simulink model "gap_generation_platoon"  (R2019a)
settings: Solver=VariableStepAuto  StartTime=0.0  StopTime=50  RelTol=1e-3
libraries: simulink x68, powerlib_meascontrol x7, autolibshared x7
(part 1 of 3)
settings Model: Creator=fvall  LastModifiedBy=fvall

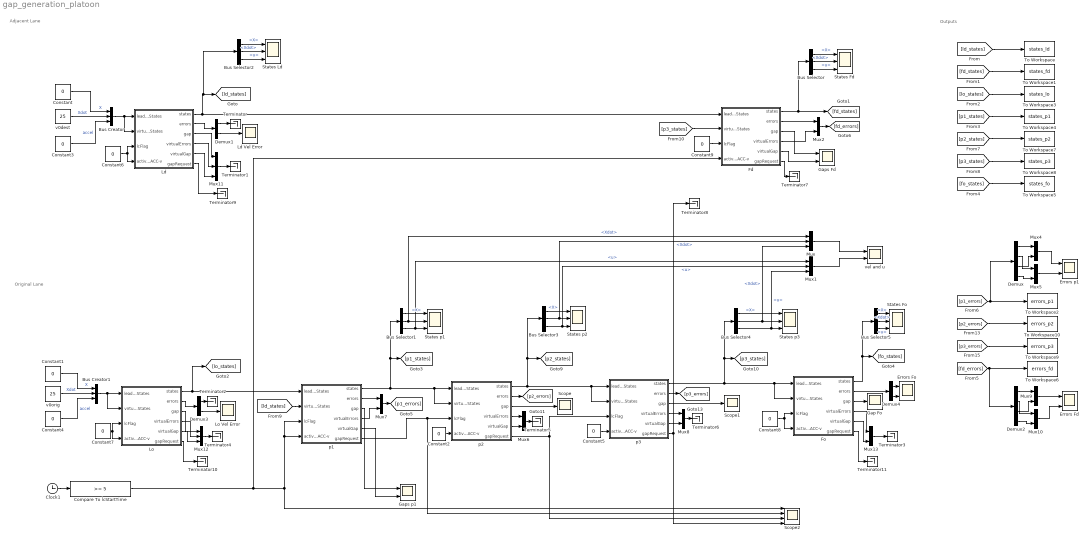
== system gap_generation_platoon ==
  note: Original Lane
  note: Adjacent Lane
  note: Outputs
  Bus Creator : BusCreator  Inputs=3
  Bus Creator1 : BusCreator  Inputs=3
  Bus Selector{,1..5} (6 alike) : BusSelector  OutputSignals=X,Xdot,u
  Clock1 : Clock
  Compare To lcStartTime : simulink/Logic and Bit Operations/Compare To Constant  relop=>=  const=5  OutDataTypeStr=boolean
  Constant{,1..9} (10 alike) : Constant  Value=0
  Demux : Demux
  Demux1 : Demux  Outputs=2
  Demux2 : Demux
  Demux3 : Demux  Outputs=2
  Demux4 : Demux  Outputs=2
  Errors Fd : Scope  NumInputPorts=2
  Errors Fo : Scope  NumInputPorts=2
  Errors p1 : Scope  NumInputPorts=2
  Fd : Subsystem  mask{m=2000, lf=2.5, lr=2.5, maxAcceleration=4, minAcceleration=-8, maxJerk=50, minJerk=-50, x0=62.7512, vx0=25, y0=3.6, h=0.63, hLc=2.215, d0=0.5004, d0Lc=0.5004, minHeadwayError=-100, maxHeadwayError=3, velFilterGain=10, Kd=1.5652, Kp=2.2775, Ki=0.75, velKi=0.5, velKp=1.5, vMin=18, hFilterGain=1, l1=-2}
      mask prompts: m "autoblks_shared:autoblkVehBody3DofLat:blkPrm_m"; lf "autoblks_shared:autoblkVehBody3DofLat:blkPrm_a"; lr "autoblks_shared:autoblkVehBody3DofLat:blkPrm_b"; maxAcceleration "Max Acceleration"; minAcceleration "Min Acceleration"; maxJerk "Max Jerk"; minJerk "Min Jerk"; x0 "autoblks_shared:autoblkVehBody3DofLat:blkPrm_X_o"; vx0 "autoblks_shared:autoblkVehBody3DofLat:blkPrm_xdot_o"; y0 "autoblks_shared:autoblkVehBody3DofLat:blkPrm_Y_o"; h "Time Headway"; hLc "Time Headway LC"; d0 "Standstill Gap"; d0Lc "Standstill Gap LC"; minHeadwayError "Min Headway Error"; maxHeadwayError "Max Headway Error"; velFilterGain "Velocity Filter Gain"; vMin "Min Gap Gen Speed"; hFilterGain "Headway filter Gain"; l1 "ACC-v Headway Error Threshold"
      mask TypeOptions m: Vehicle Body 3DOF Single Track/m
      mask TypeOptions lf: Vehicle Body 3DOF Single Track/a
      mask TypeOptions lr: Vehicle Body 3DOF Single Track/b
      mask TypeOptions x0: Vehicle Body 3DOF Single Track/X_o
      mask TypeOptions vx0: Vehicle Body 3DOF Single Track/xdot_o
      mask TypeOptions y0: Vehicle Body 3DOF Single Track/Y_o
      mask TypeOptions h: ACC/Headway error/h/Value
      mask TypeOptions hLc: ACC/Headway error/hLc/Value
      mask TypeOptions d0: ACC/Headway error/d0/Value
      mask TypeOptions d0Lc: ACC/Headway error/d0Lc/Value
      mask TypeOptions Kd: ACC/Kd/Gain
      mask TypeOptions Kp: ACC/Kp/Gain
      mask TypeOptions Ki: ACC/Ki/Gain
      mask TypeOptions velKi: ACC/velKi/Gain
      mask TypeOptions velKp: ACC/velKp/Gain
      mask TypeOptions vMin: ACC-v/vMin/Value
      mask TypeOptions hFilterGain: ACC/Headway error/hFilterGain/Gain
      mask TypeOptions l1:
      | ACC-v/Compare
      | To Constant/const
      mask DialogControl DescGroupVar Prompt: 3DOF Vehicle with ACC
      mask DialogControl DescTextVar Prompt: Vehicle with ACC. The vehicle model is Simulink's 3DOF single track vehicle body. The controller is a PID with constant headway including headway error saturation and filtered leader velocity.
      mask DialogControl ParameterGroupVar Prompt: Vehicle Parameters
      mask DialogControl m Prompt: Vehicle mass, m [kg]:
      mask DialogControl lf Prompt: Longitudinal distance from center of mass to front axle, a [m]:
      mask DialogControl lr Prompt: Longitudinal distance from center of mass to rear axle, b [m]:
      mask DialogControl x0 Prompt: Initial inertial frame longitudinal position, X_o [m]:
      mask DialogControl vx0 Prompt: Initial longitudinal velocity, xdot_o [m/s]:
      mask DialogControl y0 Prompt: Initial inertial frame lateral displacement, Y_o [m]:
      mask DialogControl Container3 Prompt: Controller Parameters
  Fo : Subsystem  mask{m=2000, lf=2.5, lr=2.5, maxAcceleration=4, minAcceleration=-8, maxJerk=50, minJerk=-50, x0=0, vx0=25, y0=0, h=0.63, hLc=2.215, d0=0.5004, d0Lc=0.5004, minHeadwayError=-100, maxHeadwayError=3, velFilterGain=10, Kd=1.5652, Kp=2.2775, Ki=0.75, velKi=0.5, velKp=1.5, vMin=18, hFilterGain=1, l1=-2}
      mask prompts: m "autoblks_shared:autoblkVehBody3DofLat:blkPrm_m"; lf "autoblks_shared:autoblkVehBody3DofLat:blkPrm_a"; lr "autoblks_shared:autoblkVehBody3DofLat:blkPrm_b"; maxAcceleration "Max Acceleration"; minAcceleration "Min Acceleration"; maxJerk "Max Jerk"; minJerk "Min Jerk"; x0 "autoblks_shared:autoblkVehBody3DofLat:blkPrm_X_o"; vx0 "autoblks_shared:autoblkVehBody3DofLat:blkPrm_xdot_o"; y0 "autoblks_shared:autoblkVehBody3DofLat:blkPrm_Y_o"; h "Time Headway"; hLc "Time Headway LC"; d0 "Standstill Gap"; d0Lc "Standstill Gap LC"; minHeadwayError "Min Headway Error"; maxHeadwayError "Max Headway Error"; velFilterGain "Velocity Filter Gain"; vMin "Min Gap Gen Speed"; hFilterGain "Headway filter Gain"; l1 "ACC-v Headway Error Threshold"
      mask TypeOptions m: Vehicle Body 3DOF Single Track/m
      mask TypeOptions lf: Vehicle Body 3DOF Single Track/a
      mask TypeOptions lr: Vehicle Body 3DOF Single Track/b
      mask TypeOptions x0: Vehicle Body 3DOF Single Track/X_o
      mask TypeOptions vx0: Vehicle Body 3DOF Single Track/xdot_o
      mask TypeOptions y0: Vehicle Body 3DOF Single Track/Y_o
      mask TypeOptions h: ACC/Headway error/h/Value
      mask TypeOptions hLc: ACC/Headway error/hLc/Value
      mask TypeOptions d0: ACC/Headway error/d0/Value
      mask TypeOptions d0Lc: ACC/Headway error/d0Lc/Value
      mask TypeOptions Kd: ACC/Kd/Gain
      mask TypeOptions Kp: ACC/Kp/Gain
      mask TypeOptions Ki: ACC/Ki/Gain
      mask TypeOptions velKi: ACC/velKi/Gain
      mask TypeOptions velKp: ACC/velKp/Gain
      mask TypeOptions vMin: ACC-v/vMin/Value
      mask TypeOptions hFilterGain: ACC/Headway error/hFilterGain/Gain
      mask TypeOptions l1:
      | ACC-v/Compare
      | To Constant/const
      mask DialogControl DescGroupVar Prompt: 3DOF Vehicle with ACC
      mask DialogControl DescTextVar Prompt: Vehicle with ACC. The vehicle model is Simulink's 3DOF single track vehicle body. The controller is a PID with constant headway including headway error saturation and filtered leader velocity.
      mask DialogControl ParameterGroupVar Prompt: Vehicle Parameters
      mask DialogControl m Prompt: Vehicle mass, m [kg]:
      mask DialogControl lf Prompt: Longitudinal distance from center of mass to front axle, a [m]:
      mask DialogControl lr Prompt: Longitudinal distance from center of mass to rear axle, b [m]:
      mask DialogControl x0 Prompt: Initial inertial frame longitudinal position, X_o [m]:
      mask DialogControl vx0 Prompt: Initial longitudinal velocity, xdot_o [m/s]:
      mask DialogControl y0 Prompt: Initial inertial frame lateral displacement, Y_o [m]:
      mask DialogControl Container3 Prompt: Controller Parameters
  Gap Fo : Scope
  Gaps Fd : Scope  NumInputPorts=2
  Gaps p1 : Scope  NumInputPorts=2
  Ld : Subsystem  mask{m=2000, lf=2.5, lr=2.5, maxAcceleration=4, minAcceleration=-8, maxJerk=50, minJerk=-50, x0=84.0016, vx0=25, y0=3.6, h=0.63, hLc=1.9025, d0=0.5004, d0Lc=0.5004, minHeadwayError=-100, maxHeadwayError=3, velFilterGain=10, Kd=1.5652, Kp=2.2775, Ki=0.75, velKi=0.5, velKp=1.5, vMin=18, hFilterGain=1, l1=-2}
      mask prompts: m "autoblks_shared:autoblkVehBody3DofLat:blkPrm_m"; lf "autoblks_shared:autoblkVehBody3DofLat:blkPrm_a"; lr "autoblks_shared:autoblkVehBody3DofLat:blkPrm_b"; maxAcceleration "Max Acceleration"; minAcceleration "Min Acceleration"; maxJerk "Max Jerk"; minJerk "Min Jerk"; x0 "autoblks_shared:autoblkVehBody3DofLat:blkPrm_X_o"; vx0 "autoblks_shared:autoblkVehBody3DofLat:blkPrm_xdot_o"; y0 "autoblks_shared:autoblkVehBody3DofLat:blkPrm_Y_o"; h "Time Headway"; hLc "Time Headway LC"; d0 "Standstill Gap"; d0Lc "Standstill Gap LC"; minHeadwayError "Min Headway Error"; maxHeadwayError "Max Headway Error"; velFilterGain "Velocity Filter Gain"; vMin "Min Gap Gen Speed"; hFilterGain "Headway filter Gain"; l1 "ACC-v Headway Error Threshold"
      mask TypeOptions m: Vehicle Body 3DOF Single Track/m
      mask TypeOptions lf: Vehicle Body 3DOF Single Track/a
      mask TypeOptions lr: Vehicle Body 3DOF Single Track/b
      mask TypeOptions x0: Vehicle Body 3DOF Single Track/X_o
      mask TypeOptions vx0: Vehicle Body 3DOF Single Track/xdot_o
      mask TypeOptions y0: Vehicle Body 3DOF Single Track/Y_o
      mask TypeOptions h: ACC/Headway error/h/Value
      mask TypeOptions hLc: ACC/Headway error/hLc/Value
      mask TypeOptions d0: ACC/Headway error/d0/Value
      mask TypeOptions d0Lc: ACC/Headway error/d0Lc/Value
      mask TypeOptions Kd: ACC/Kd/Gain
      mask TypeOptions Kp: ACC/Kp/Gain
      mask TypeOptions Ki: ACC/Ki/Gain
      mask TypeOptions velKi: ACC/velKi/Gain
      mask TypeOptions velKp: ACC/velKp/Gain
      mask TypeOptions vMin: ACC-v/vMin/Value
      mask TypeOptions hFilterGain: ACC/Headway error/hFilterGain/Gain
      mask TypeOptions l1:
      | ACC-v/Compare
      | To Constant/const
      mask DialogControl DescGroupVar Prompt: 3DOF Vehicle with ACC
      mask DialogControl DescTextVar Prompt: Vehicle with ACC. The vehicle model is Simulink's 3DOF single track vehicle body. The controller is a PID with constant headway including headway error saturation and filtered leader velocity.
      mask DialogControl ParameterGroupVar Prompt: Vehicle Parameters
      mask DialogControl m Prompt: Vehicle mass, m [kg]:
      mask DialogControl lf Prompt: Longitudinal distance from center of mass to front axle, a [m]:
      mask DialogControl lr Prompt: Longitudinal distance from center of mass to rear axle, b [m]:
      mask DialogControl x0 Prompt: Initial inertial frame longitudinal position, X_o [m]:
      mask DialogControl vx0 Prompt: Initial longitudinal velocity, xdot_o [m/s]:
      mask DialogControl y0 Prompt: Initial inertial frame lateral displacement, Y_o [m]:
      mask DialogControl Container3 Prompt: Controller Parameters
  Ld Vel Error : Scope
  Lo : Subsystem  mask{m=2000, lf=2.5, lr=2.5, maxAcceleration=4, minAcceleration=-8, maxJerk=50, minJerk=-50, x0=85.0016, vx0=25, y0=0, h=0.63, hLc=1.9025, d0=0.5004, d0Lc=0.5004, minHeadwayError=-100, maxHeadwayError=3, velFilterGain=10, Kd=1.5652, Kp=2.2775, Ki=0.75, velKi=0.5, velKp=1.5, vMin=18, hFilterGain=1, l1=-2}
      mask prompts: m "autoblks_shared:autoblkVehBody3DofLat:blkPrm_m"; lf "autoblks_shared:autoblkVehBody3DofLat:blkPrm_a"; lr "autoblks_shared:autoblkVehBody3DofLat:blkPrm_b"; maxAcceleration "Max Acceleration"; minAcceleration "Min Acceleration"; maxJerk "Max Jerk"; minJerk "Min Jerk"; x0 "autoblks_shared:autoblkVehBody3DofLat:blkPrm_X_o"; vx0 "autoblks_shared:autoblkVehBody3DofLat:blkPrm_xdot_o"; y0 "autoblks_shared:autoblkVehBody3DofLat:blkPrm_Y_o"; h "Time Headway"; hLc "Time Headway LC"; d0 "Standstill Gap"; d0Lc "Standstill Gap LC"; minHeadwayError "Min Headway Error"; maxHeadwayError "Max Headway Error"; velFilterGain "Velocity Filter Gain"; vMin "Min Gap Gen Speed"; hFilterGain "Headway filter Gain"; l1 "ACC-v Headway Error Threshold"
      mask TypeOptions m: Vehicle Body 3DOF Single Track/m
      mask TypeOptions lf: Vehicle Body 3DOF Single Track/a
      mask TypeOptions lr: Vehicle Body 3DOF Single Track/b
      mask TypeOptions x0: Vehicle Body 3DOF Single Track/X_o
      mask TypeOptions vx0: Vehicle Body 3DOF Single Track/xdot_o
      mask TypeOptions y0: Vehicle Body 3DOF Single Track/Y_o
      mask TypeOptions h: ACC/Headway error/h/Value
      mask TypeOptions hLc: ACC/Headway error/hLc/Value
      mask TypeOptions d0: ACC/Headway error/d0/Value
      mask TypeOptions d0Lc: ACC/Headway error/d0Lc/Value
      mask TypeOptions Kd: ACC/Kd/Gain
      mask TypeOptions Kp: ACC/Kp/Gain
      mask TypeOptions Ki: ACC/Ki/Gain
      mask TypeOptions velKi: ACC/velKi/Gain
      mask TypeOptions velKp: ACC/velKp/Gain
      mask TypeOptions vMin: ACC-v/vMin/Value
      mask TypeOptions hFilterGain: ACC/Headway error/hFilterGain/Gain
      mask TypeOptions l1:
      | ACC-v/Compare
      | To Constant/const
      mask DialogControl DescGroupVar Prompt: 3DOF Vehicle with ACC
      mask DialogControl DescTextVar Prompt: Vehicle with ACC. The vehicle model is Simulink's 3DOF single track vehicle body. The controller is a PID with constant headway including headway error saturation and filtered leader velocity.
      mask DialogControl ParameterGroupVar Prompt: Vehicle Parameters
      mask DialogControl m Prompt: Vehicle mass, m [kg]:
      mask DialogControl lf Prompt: Longitudinal distance from center of mass to front axle, a [m]:
      mask DialogControl lr Prompt: Longitudinal distance from center of mass to rear axle, b [m]:
      mask DialogControl x0 Prompt: Initial inertial frame longitudinal position, X_o [m]:
      mask DialogControl vx0 Prompt: Initial longitudinal velocity, xdot_o [m/s]:
      mask DialogControl y0 Prompt: Initial inertial frame lateral displacement, Y_o [m]:
      mask DialogControl Container3 Prompt: Controller Parameters
  Lo Vel Error : Scope
  Mux{,1,11..12} (4 alike) : Mux  Inputs=3
  Mux{2,4..10,13} (9 alike) : Mux  Inputs=2
  Scope : Scope
  Scope1 : Scope
  Scope2 : Scope  NumInputPorts=4
  States Fd : Scope  NumInputPorts=3
  States Fo : Scope  NumInputPorts=3
  States Ld : Scope  NumInputPorts=3
  States p1 : Scope  NumInputPorts=3
  States p2 : Scope  NumInputPorts=3
  States p3 : Scope  NumInputPorts=3
  Terminator{,1..11} (12 alike) : Terminator
  To Workspace : ToWorkspace  VariableName=states_ld  SampleTime=-1
  To Workspace1 : ToWorkspace  VariableName=states_fd  SampleTime=-1
  To Workspace10 : ToWorkspace  VariableName=errors_p2  SampleTime=-1
  To Workspace2 : ToWorkspace  VariableName=errors_p1  SampleTime=-1
  To Workspace3 : ToWorkspace  VariableName=states_lo  SampleTime=-1
  To Workspace4 : ToWorkspace  VariableName=states_p1  SampleTime=-1
  To Workspace5 : ToWorkspace  VariableName=states_fo  SampleTime=-1
  To Workspace6 : ToWorkspace  VariableName=errors_fd  SampleTime=-1
  To Workspace7 : ToWorkspace  VariableName=states_p2  SampleTime=-1
  To Workspace8 : ToWorkspace  VariableName=states_p3  SampleTime=-1
  To Workspace9 : ToWorkspace  VariableName=errors_p3  SampleTime=-1
  p1 : Subsystem  mask{m=2000, lf=2.5, lr=2.5, maxAcceleration=4, minAcceleration=-8, maxJerk=50, minJerk=-50, x0=63.7512, vx0=25, y0=0, h=0.63, hLc=2.215, d0=0.5004, d0Lc=0.5004, minHeadwayError=-100, maxHeadwayError=3, velFilterGain=10, Kd=1.5652, Kp=2.2775, Ki=0.75, velKi=0.5, velKp=1.5, vMin=18, hFilterGain=1, l1=-2}
      mask prompts: m "autoblks_shared:autoblkVehBody3DofLat:blkPrm_m"; lf "autoblks_shared:autoblkVehBody3DofLat:blkPrm_a"; lr "autoblks_shared:autoblkVehBody3DofLat:blkPrm_b"; maxAcceleration "Max Acceleration"; minAcceleration "Min Acceleration"; maxJerk "Max Jerk"; minJerk "Min Jerk"; x0 "autoblks_shared:autoblkVehBody3DofLat:blkPrm_X_o"; vx0 "autoblks_shared:autoblkVehBody3DofLat:blkPrm_xdot_o"; y0 "autoblks_shared:autoblkVehBody3DofLat:blkPrm_Y_o"; h "Time Headway"; hLc "Time Headway LC"; d0 "Standstill Gap"; d0Lc "Standstill Gap LC"; minHeadwayError "Min Headway Error"; maxHeadwayError "Max Headway Error"; velFilterGain "Velocity Filter Gain"; vMin "Min Gap Gen Speed"; hFilterGain "Headway filter Gain"; l1 "ACC-v Headway Error Threshold"
      mask TypeOptions m: Vehicle Body 3DOF Single Track/m
      mask TypeOptions lf: Vehicle Body 3DOF Single Track/a
      mask TypeOptions lr: Vehicle Body 3DOF Single Track/b
      mask TypeOptions x0: Vehicle Body 3DOF Single Track/X_o
      mask TypeOptions vx0: Vehicle Body 3DOF Single Track/xdot_o
      mask TypeOptions y0: Vehicle Body 3DOF Single Track/Y_o
      mask TypeOptions h: ACC/Headway error/h/Value
      mask TypeOptions hLc: ACC/Headway error/hLc/Value
      mask TypeOptions d0: ACC/Headway error/d0/Value
      mask TypeOptions d0Lc: ACC/Headway error/d0Lc/Value
      mask TypeOptions Kd: ACC/Kd/Gain
      mask TypeOptions Kp: ACC/Kp/Gain
      mask TypeOptions Ki: ACC/Ki/Gain
      mask TypeOptions velKi: ACC/velKi/Gain
      mask TypeOptions velKp: ACC/velKp/Gain
      mask TypeOptions vMin: ACC-v/vMin/Value
      mask TypeOptions hFilterGain: ACC/Headway error/hFilterGain/Gain
      mask TypeOptions l1:
      | ACC-v/Compare
      | To Constant/const
      mask DialogControl DescGroupVar Prompt: 3DOF Vehicle with ACC
      mask DialogControl DescTextVar Prompt: Vehicle with ACC. The vehicle model is Simulink's 3DOF single track vehicle body. The controller is a PID with constant headway including headway error saturation and filtered leader velocity.
      mask DialogControl ParameterGroupVar Prompt: Vehicle Parameters
      mask DialogControl m Prompt: Vehicle mass, m [kg]:
      mask DialogControl lf Prompt: Longitudinal distance from center of mass to front axle, a [m]:
      mask DialogControl lr Prompt: Longitudinal distance from center of mass to rear axle, b [m]:
      mask DialogControl x0 Prompt: Initial inertial frame longitudinal position, X_o [m]:
      mask DialogControl vx0 Prompt: Initial longitudinal velocity, xdot_o [m/s]:
      mask DialogControl y0 Prompt: Initial inertial frame lateral displacement, Y_o [m]:
      mask DialogControl Container3 Prompt: Controller Parameters
  p2 : Subsystem  mask{m=2000, lf=2.5, lr=2.5, maxAcceleration=4, minAcceleration=-8, maxJerk=50, minJerk=-50, x0=42.5008, vx0=25, y0=0, h=0.63, hLc=2.215, d0=0.5004, d0Lc=0.5004, minHeadwayError=-100, maxHeadwayError=3, velFilterGain=10, Kd=1.5652, Kp=2.2775, Ki=0.75, velKi=0.5, velKp=1.5, vMin=18, hFilterGain=1, l1=-2}
      mask prompts: m "autoblks_shared:autoblkVehBody3DofLat:blkPrm_m"; lf "autoblks_shared:autoblkVehBody3DofLat:blkPrm_a"; lr "autoblks_shared:autoblkVehBody3DofLat:blkPrm_b"; maxAcceleration "Max Acceleration"; minAcceleration "Min Acceleration"; maxJerk "Max Jerk"; minJerk "Min Jerk"; x0 "autoblks_shared:autoblkVehBody3DofLat:blkPrm_X_o"; vx0 "autoblks_shared:autoblkVehBody3DofLat:blkPrm_xdot_o"; y0 "autoblks_shared:autoblkVehBody3DofLat:blkPrm_Y_o"; h "Time Headway"; hLc "Time Headway LC"; d0 "Standstill Gap"; d0Lc "Standstill Gap LC"; minHeadwayError "Min Headway Error"; maxHeadwayError "Max Headway Error"; velFilterGain "Velocity Filter Gain"; vMin "Min Gap Gen Speed"; hFilterGain "Headway filter Gain"; l1 "ACC-v Headway Error Threshold"
      mask TypeOptions m: Vehicle Body 3DOF Single Track/m
      mask TypeOptions lf: Vehicle Body 3DOF Single Track/a
      mask TypeOptions lr: Vehicle Body 3DOF Single Track/b
      mask TypeOptions x0: Vehicle Body 3DOF Single Track/X_o
      mask TypeOptions vx0: Vehicle Body 3DOF Single Track/xdot_o
      mask TypeOptions y0: Vehicle Body 3DOF Single Track/Y_o
      mask TypeOptions h: ACC/Headway error/h/Value
      mask TypeOptions hLc: ACC/Headway error/hLc/Value
      mask TypeOptions d0: ACC/Headway error/d0/Value
      mask TypeOptions d0Lc: ACC/Headway error/d0Lc/Value
      mask TypeOptions Kd: ACC/Kd/Gain
      mask TypeOptions Kp: ACC/Kp/Gain
      mask TypeOptions Ki: ACC/Ki/Gain
      mask TypeOptions velKi: ACC/velKi/Gain
      mask TypeOptions velKp: ACC/velKp/Gain
      mask TypeOptions vMin: ACC-v/vMin/Value
      mask TypeOptions hFilterGain: ACC/Headway error/hFilterGain/Gain
      mask TypeOptions l1:
      | ACC-v/Compare
      | To Constant/const
      mask DialogControl DescGroupVar Prompt: 3DOF Vehicle with ACC
      mask DialogControl DescTextVar Prompt: Vehicle with ACC. The vehicle model is Simulink's 3DOF single track vehicle body. The controller is a PID with constant headway including headway error saturation and filtered leader velocity.
      mask DialogControl ParameterGroupVar Prompt: Vehicle Parameters
      mask DialogControl m Prompt: Vehicle mass, m [kg]:
      mask DialogControl lf Prompt: Longitudinal distance from center of mass to front axle, a [m]:
      mask DialogControl lr Prompt: Longitudinal distance from center of mass to rear axle, b [m]:
      mask DialogControl x0 Prompt: Initial inertial frame longitudinal position, X_o [m]:
      mask DialogControl vx0 Prompt: Initial longitudinal velocity, xdot_o [m/s]:
      mask DialogControl y0 Prompt: Initial inertial frame lateral displacement, Y_o [m]:
      mask DialogControl Container3 Prompt: Controller Parameters
  p3 : Subsystem  mask{m=2000, lf=2.5, lr=2.5, maxAcceleration=4, minAcceleration=-8, maxJerk=50, minJerk=-50, x0=21.2504, vx0=25, y0=0, h=0.63, hLc=2.215, d0=0.5004, d0Lc=0.5004, minHeadwayError=-100, maxHeadwayError=3, velFilterGain=10, Kd=1.5652, Kp=2.2775, Ki=0.75, velKi=0.5, velKp=1.5, vMin=18, hFilterGain=1, l1=-2}
      mask prompts: m "autoblks_shared:autoblkVehBody3DofLat:blkPrm_m"; lf "autoblks_shared:autoblkVehBody3DofLat:blkPrm_a"; lr "autoblks_shared:autoblkVehBody3DofLat:blkPrm_b"; maxAcceleration "Max Acceleration"; minAcceleration "Min Acceleration"; maxJerk "Max Jerk"; minJerk "Min Jerk"; x0 "autoblks_shared:autoblkVehBody3DofLat:blkPrm_X_o"; vx0 "autoblks_shared:autoblkVehBody3DofLat:blkPrm_xdot_o"; y0 "autoblks_shared:autoblkVehBody3DofLat:blkPrm_Y_o"; h "Time Headway"; hLc "Time Headway LC"; d0 "Standstill Gap"; d0Lc "Standstill Gap LC"; minHeadwayError "Min Headway Error"; maxHeadwayError "Max Headway Error"; velFilterGain "Velocity Filter Gain"; vMin "Min Gap Gen Speed"; hFilterGain "Headway filter Gain"; l1 "ACC-v Headway Error Threshold"
      mask TypeOptions m: Vehicle Body 3DOF Single Track/m
      mask TypeOptions lf: Vehicle Body 3DOF Single Track/a
      mask TypeOptions lr: Vehicle Body 3DOF Single Track/b
      mask TypeOptions x0: Vehicle Body 3DOF Single Track/X_o
      mask TypeOptions vx0: Vehicle Body 3DOF Single Track/xdot_o
      mask TypeOptions y0: Vehicle Body 3DOF Single Track/Y_o
      mask TypeOptions h: ACC/Headway error/h/Value
      mask TypeOptions hLc: ACC/Headway error/hLc/Value
      mask TypeOptions d0: ACC/Headway error/d0/Value
      mask TypeOptions d0Lc: ACC/Headway error/d0Lc/Value
      mask TypeOptions Kd: ACC/Kd/Gain
      mask TypeOptions Kp: ACC/Kp/Gain
      mask TypeOptions Ki: ACC/Ki/Gain
      mask TypeOptions velKi: ACC/velKi/Gain
      mask TypeOptions velKp: ACC/velKp/Gain
      mask TypeOptions vMin: ACC-v/vMin/Value
      mask TypeOptions hFilterGain: ACC/Headway error/hFilterGain/Gain
      mask TypeOptions l1:
      | ACC-v/Compare
      | To Constant/const
      mask DialogControl DescGroupVar Prompt: 3DOF Vehicle with ACC
      mask DialogControl DescTextVar Prompt: Vehicle with ACC. The vehicle model is Simulink's 3DOF single track vehicle body. The controller is a PID with constant headway including headway error saturation and filtered leader velocity.
      mask DialogControl ParameterGroupVar Prompt: Vehicle Parameters
      mask DialogControl m Prompt: Vehicle mass, m [kg]:
      mask DialogControl lf Prompt: Longitudinal distance from center of mass to front axle, a [m]:
      mask DialogControl lr Prompt: Longitudinal distance from center of mass to rear axle, b [m]:
      mask DialogControl x0 Prompt: Initial inertial frame longitudinal position, X_o [m]:
      mask DialogControl vx0 Prompt: Initial longitudinal velocity, xdot_o [m/s]:
      mask DialogControl y0 Prompt: Initial inertial frame lateral displacement, Y_o [m]:
      mask DialogControl Container3 Prompt: Controller Parameters
  v0dest : Constant  Value=25
  v0orig : Constant  Value=25
  vel and u : Scope  NumInputPorts=2
  wires:
  Clock1/1 -> Compare To lcStartTime/1
  Bus Selector3/3 -> Mux1/2, States p2/3  "<u>"
  Bus Selector3/2 -> Mux/2, States p2/2  "<Xdot>"
  Bus Selector3/1 -> States p2/1  "<X>"
  p2/1(states) -> p3/1(leaderStates), p3/2(virtualLeaderStates), [p2_states], Bus Selector3/1
  Bus Selector4/3 -> Mux1/3, States p3/3  "<u>"
  Bus Selector4/2 -> States p3/2, Mux/3  "<Xdot>"
  Bus Selector4/1 -> States p3/1  "<X>"
  p2/2(errors) -> [p2_errors]
  p3/2(errors) -> [p3_errors]
  [p2_errors] -> To Workspace10/1
  [p3_errors] -> To Workspace9/1
  Ld/2(errors) -> Demux1/1
  Bus Selector2/3 -> States Ld/3  "<u>"
  Fd/6(gapRequest) -> Terminator7/1
  Fd/4(virtualErrors) -> Mux2/2
  Fd/5(virtualGap) -> Gaps Fd/2
  Fd/1(states) -> Bus Selector/1, [fd_states]
  Ld/3(gap) -> Mux11/1
  Fd/3(gap) -> Gaps Fd/1
  Mux11/1 -> Terminator1/1
  Fd/2(errors) -> Mux2/1
  Demux1/2 -> Ld Vel Error/1
  Bus Selector2/2 -> States Ld/2  "<Xdot>"
  Bus Selector2/1 -> States Ld/1  "<X>"
  Ld/6(gapRequest) -> Terminator9/1
  Bus Selector/1 -> States Fd/1  "<X>"
  [p3_states] -> Fd/2(virtualLeaderStates)
  Constant9/1 -> Fd/3(lcFlag)
  Ld/5(virtualGap) -> Mux11/3
  Bus Selector/3 -> States Fd/3  "<u>"
  Constant6/1 -> Ld/3(lcFlag), Ld/4(activate ACC-v)
  Ld/4(virtualErrors) -> Mux11/2
  Bus Selector/2 -> States Fd/2  "<Xdot>"
  Ld/1(states) -> Fd/1(leaderStates), Bus Selector2/1, [ld_states]
  v0dest/1 -> Bus Creator/2  "Xdot"
  Constant3/1 -> Bus Creator/3  "accel"
  Mux2/1 -> [fd_errors]
  Constant/1 -> Bus Creator/1  "X"
  Demux1/1 -> Terminator/1
  Bus Creator/1 -> Ld/1(leaderStates), Ld/2(virtualLeaderStates)
  Lo/5(virtualGap) -> Mux12/3
  Lo/2(errors) -> Demux3/1
  Mux12/1 -> Terminator4/1
  Lo/3(gap) -> Mux12/1
  Lo/1(states) -> p1/1(leaderStates), [lo_states]
  Lo/6(gapRequest) -> Terminator10/1
  Demux3/1 -> Terminator2/1
  Bus Creator1/1 -> Lo/2(virtualLeaderStates), Lo/1(leaderStates)
  Lo/4(virtualErrors) -> Mux12/2
  Constant7/1 -> Lo/3(lcFlag), Lo/4(activate ACC-v)
  v0orig/1 -> Bus Creator1/2  "Xdot"
  Constant4/1 -> Bus Creator1/3  "accel"
  Constant1/1 -> Bus Creator1/1  "X"
  Demux3/2 -> Lo Vel Error/1
  Mux13/1 -> Terminator3/1
  Fo/2(errors) -> Demux4/1
  Fo/4(virtualErrors) -> Mux13/1
  Fo/6(gapRequest) -> Terminator11/1
  Fo/3(gap) -> Gap Fo/1
  Demux4/2 -> Errors Fo/2
  Constant8/1 -> Fo/3(lcFlag), Fo/4(activate ACC-v)
  Demux4/1 -> Errors Fo/1
  Fo/1(states) -> Bus Selector5/1, [fo_states]
  p3/1(states) -> Bus Selector4/1, [p3_states], Fo/1(leaderStates), Fo/2(virtualLeaderStates)
  Fo/5(virtualGap) -> Mux13/2
  p1/4(virtualErrors) -> Mux7/2
  p1/1(states) -> Bus Selector1/1, [p1_states], p2/2(virtualLeaderStates), p2/1(leaderStates)
  Bus Selector1/2 -> States p1/2, Mux/1  "<Xdot>"
  p1/5(virtualGap) -> Gaps p1/2
  Mux7/1 -> [p1_errors]
  Bus Selector1/1 -> States p1/1  "<X>"
  Compare To lcStartTime/1 -> Fd/4(activate ACC-v), Scope2/1, p1/3(lcFlag), p1/4(activate ACC-v)
  Bus Selector1/3 -> Mux1/1, States p1/3  "<u>"
  p1/2(errors) -> Mux7/1
  p1/3(gap) -> Gaps p1/1
  [ld_states] -> p1/2(virtualLeaderStates)
  p1/6(gapRequest) -> p2/3(lcFlag), Scope2/2
  p2/6(gapRequest) -> p3/3(lcFlag), Scope2/3
  p3/6(gapRequest) -> Terminator8/1, Scope2/4
  p2/4(virtualErrors) -> Mux6/1
  p2/5(virtualGap) -> Mux6/2
  Mux6/1 -> Terminator5/1
  p3/4(virtualErrors) -> Mux8/1
  Mux8/1 -> Terminator6/1
  p3/5(virtualGap) -> Mux8/2
  p2/3(gap) -> Scope/1
  p3/3(gap) -> Scope1/1
  [fd_states] -> To Workspace1/1
  [lo_states] -> To Workspace3/1
  Mux10/1 -> Errors Fd/2
  Mux4/1 -> Errors p1/1
  Demux/2 -> Mux5/1
  Mux9/1 -> Errors Fd/1
  Demux/3 -> Mux4/2
  Demux/1 -> Mux4/1
  Mux5/1 -> Errors p1/2
  Demux2/2 -> Mux10/1
  Demux2/3 -> Mux9/2
  [p1_errors] -> To Workspace2/1, Demux/1
  [fd_errors] -> Demux2/1, To Workspace6/1
  [p1_states] -> To Workspace4/1
  Demux2/4 -> Mux10/2
  [ld_states] -> To Workspace/1
  Demux/4 -> Mux5/2
  [fo_states] -> To Workspace5/1
  Demux2/1 -> Mux9/1
  [p2_states] -> To Workspace7/1
  [p3_states] -> To Workspace8/1
  Mux/1 -> vel and u/1
  Mux1/1 -> vel and u/2
  Constant2/1 -> p2/4(activate ACC-v)
  Constant5/1 -> p3/4(activate ACC-v)
  Bus Selector5/1 -> States Fo/1  "<X>"
  Bus Selector5/2 -> States Fo/2  "<Xdot>"
  Bus Selector5/3 -> States Fo/3  "<u>"

== system gap_generation_platoon/Fd ==
  leaderStates : Inport
  virtualLeaderStates : Inport  Port=2
  lcFlag : Inport  Port=3
  activate ACC-v : Inport  Port=4
  ACC : Subsystem
  ACC-v : Subsystem
  AND : Logic  Inputs=3  IconShape=distinctive  AllPortsSameDT=off  OutDataTypeStr=boolean
  Abs : Abs
  Abs1 : Abs  ZeroCross=off
  Bus Creator : BusCreator  Inputs=4
  Bus Selector : BusSelector  OutputSignals=InertFrm.RearAxl.Disp.X,InertFrm.RearAxl.Disp.Y,InertFrm.RearAxl.Vel.Xdot
  Compare To Constant : simulink/Logic and Bit Operations/Compare To Constant  relop=<=  const=0.5  OutDataTypeStr=boolean
  Compare To Constant1 : simulink/Logic and Bit Operations/Compare To Constant  relop=<=  const=0.5  OutDataTypeStr=boolean
  Constant : Constant  Value=0
  Constant1 : Constant  Value=maxAcceleration+1
  Gain : Gain  Gain=m/2
  Min : MinMax  Inputs=2
  Mux1 : Mux  Inputs=6
  On Delay : powerlib_meascontrol/Logic/On Delay  DelayType=On delay  delay=1  ic=0  Ts=0
      settings: SourceProductName=Simscape Electrical
  Scope : Scope  NumInputPorts=2
  Scope1 : Scope  NumInputPorts=3
  Signal Specification : SignalSpecification  Dimensions=1
  Switch : Switch  Criteria=u2 > Threshold
  Terminator : Terminator
  Transport Delay : TransportDelay
  Triggered Subsystem : Subsystem  TreatAsAtomicUnit=on
  Vehicle Body 3DOF Single Track : autolibshared/Vehicle Body 3DOF Single Track  trackMode=Single (bicycle)  inputMode=External longitudinal forces  frontSteerMode=on  rearSteerMode=off  windMode=off  muMode=off  extFMode=off  extMMode=off  extXo=off  extpsio=off  extxdoto=off  extro=off  extYo=off  extTamb=off  extydoto=off  aMode=2  NF=2  NR=2  m=m  a=lf  b=lr  h=0.35  X_o=x0  xdot_o=vx0  CalphaMode=off  sigmaMode=on  d=0  w=[1.4,1.4]  Cy_f=12e3  Cy_r=11e3  sigma_f=.1  sigma_r=.1  alpha_f_brk=[-.1 .1]  Cy_f_data=[-9e3 9e3]  alpha_r_brk=[-.1 .1]  Cy_r_data=[-9e3 9e3]  Y_o=y0  ydot_o=0  Izz=4000  psi_o=0  r_o=0  Af=2  Cd=.3  Cl=.1  Cpm=.1  beta_w=[0:0.01:0.3]  Cs=[0:0.03:0.9]  Cym=[0:0.01:0.3]  Pabs=101325  Tair=273  g=9.81  mu=1  xdot_tol=.01  Fznom=5000  Fxtire_sat=7e4  Fytire_sat=7e4  longOff=0  latOff=0  vertOff=0  wrapAng=off
      settings: SourceProductName=Powertrain Blockset  SourceProductBaseCode=PW
  states : Outport
  errors : Outport  Port=2
  gap : Outport  Port=3
  virtualErrors : Outport  Port=4
  virtualGap : Outport  Port=5
  gapRequest : Outport  Port=6
  wires:
  Bus Selector/3 -> Bus Creator/3  "<Xdot>"
  Bus Selector/1 -> Bus Creator/1  "<X>"
  Min/1 -> Scope1/3, Signal Specification/1  "u"
  ACC/1(u) -> Scope1/1, Min/1  "acc"
  Gain/1 -> Vehicle Body 3DOF Single Track/3, Vehicle Body 3DOF Single Track/2
  Constant/1 -> Vehicle Body 3DOF Single Track/1
  Vehicle Body 3DOF Single Track/1 -> Bus Selector/1
  Vehicle Body 3DOF Single Track/4 -> Mux1/3
  Vehicle Body 3DOF Single Track/3 -> Mux1/2
  Vehicle Body 3DOF Single Track/2 -> Mux1/1
  Vehicle Body 3DOF Single Track/5 -> Mux1/4
  Vehicle Body 3DOF Single Track/6 -> Mux1/5
  Vehicle Body 3DOF Single Track/7 -> Mux1/6
  Mux1/1 -> Terminator/1
  ACC/3(gap) -> gap/1
  Bus Creator/1 -> ACC/1(currentStates), ACC-v/1(currentStates), states/1
  leaderStates/1 -> ACC/2(leaderStates)
  virtualLeaderStates/1 -> ACC-v/2(leaderStates)
  ACC/2(errors) -> errors/1
  lcFlag/1 -> ACC-v/4(lcFlag), On Delay/1, ACC/3(lcFlag)
  Switch/1 -> Scope1/2, Min/2  "acc-v"
  ACC-v/1(u) -> Switch/1
  ACC-v/2(errors) -> virtualErrors/1
  ACC-v/3(gap) -> virtualGap/1
  Bus Selector/2 -> Bus Creator/2  "<Y>"
  Signal Specification/1 -> Transport Delay/1, Abs1/1, Bus Creator/4, Gain/1
  activate ACC-v/1 -> ACC-v/3(activate), Switch/2
  Constant1/1 -> Switch/3
  AND/1 -> Triggered Subsystem/Trigger
  Compare To Constant1/1 -> Scope/1, AND/1
  On Delay/1 -> AND/3, Triggered Subsystem/1(In1)
  Triggered Subsystem/1(Out1) -> gapRequest/1, Scope/2
  Compare To Constant/1 -> AND/2
  Transport Delay/1 -> Abs/1
  Abs/1 -> Compare To Constant/1
  Abs1/1 -> Compare To Constant1/1

== system gap_generation_platoon/Fo ==
  leaderStates : Inport
  virtualLeaderStates : Inport  Port=2
  lcFlag : Inport  Port=3
  activate ACC-v : Inport  Port=4
  ACC : Subsystem
  ACC-v : Subsystem
  AND : Logic  Inputs=3  IconShape=distinctive  AllPortsSameDT=off  OutDataTypeStr=boolean
  Abs : Abs
  Abs1 : Abs  ZeroCross=off
  Bus Creator : BusCreator  Inputs=4
  Bus Selector : BusSelector  OutputSignals=InertFrm.RearAxl.Disp.X,InertFrm.RearAxl.Disp.Y,InertFrm.RearAxl.Vel.Xdot
  Compare To Constant : simulink/Logic and Bit Operations/Compare To Constant  relop=<=  const=0.5  OutDataTypeStr=boolean
  Compare To Constant1 : simulink/Logic and Bit Operations/Compare To Constant  relop=<=  const=0.5  OutDataTypeStr=boolean
  Constant : Constant  Value=0
  Constant1 : Constant  Value=maxAcceleration+1
  Gain : Gain  Gain=m/2
  Min : MinMax  Inputs=2
  Mux1 : Mux  Inputs=6
  On Delay : powerlib_meascontrol/Logic/On Delay  DelayType=On delay  delay=1  ic=0  Ts=0
      settings: SourceProductName=Simscape Electrical
  Scope : Scope  NumInputPorts=2
  Scope1 : Scope  NumInputPorts=3
  Signal Specification : SignalSpecification  Dimensions=1
  Switch : Switch  Criteria=u2 > Threshold
  Terminator : Terminator
  Transport Delay : TransportDelay
  Triggered Subsystem : Subsystem  TreatAsAtomicUnit=on
  Vehicle Body 3DOF Single Track : autolibshared/Vehicle Body 3DOF Single Track  trackMode=Single (bicycle)  inputMode=External longitudinal forces  frontSteerMode=on  rearSteerMode=off  windMode=off  muMode=off  extFMode=off  extMMode=off  extXo=off  extpsio=off  extxdoto=off  extro=off  extYo=off  extTamb=off  extydoto=off  aMode=2  NF=2  NR=2  m=m  a=lf  b=lr  h=0.35  X_o=x0  xdot_o=vx0  CalphaMode=off  sigmaMode=on  d=0  w=[1.4,1.4]  Cy_f=12e3  Cy_r=11e3  sigma_f=.1  sigma_r=.1  alpha_f_brk=[-.1 .1]  Cy_f_data=[-9e3 9e3]  alpha_r_brk=[-.1 .1]  Cy_r_data=[-9e3 9e3]  Y_o=y0  ydot_o=0  Izz=4000  psi_o=0  r_o=0  Af=2  Cd=.3  Cl=.1  Cpm=.1  beta_w=[0:0.01:0.3]  Cs=[0:0.03:0.9]  Cym=[0:0.01:0.3]  Pabs=101325  Tair=273  g=9.81  mu=1  xdot_tol=.01  Fznom=5000  Fxtire_sat=7e4  Fytire_sat=7e4  longOff=0  latOff=0  vertOff=0  wrapAng=off
      settings: SourceProductName=Powertrain Blockset  SourceProductBaseCode=PW
  states : Outport
  errors : Outport  Port=2
  gap : Outport  Port=3
  virtualErrors : Outport  Port=4
  virtualGap : Outport  Port=5
  gapRequest : Outport  Port=6
  wires:
  Abs1/1 -> Compare To Constant1/1
  Abs/1 -> Compare To Constant/1
  Transport Delay/1 -> Abs/1
  Compare To Constant/1 -> AND/2
  Triggered Subsystem/1(Out1) -> Scope/2, gapRequest/1
  On Delay/1 -> Triggered Subsystem/1(In1), AND/3
  Compare To Constant1/1 -> AND/1, Scope/1
  AND/1 -> Triggered Subsystem/Trigger
  Constant1/1 -> Switch/3
  activate ACC-v/1 -> Switch/2, ACC-v/3(activate)
  Signal Specification/1 -> Gain/1, Bus Creator/4, Abs1/1, Transport Delay/1
  Bus Selector/2 -> Bus Creator/2  "<Y>"
  ACC-v/3(gap) -> virtualGap/1
  ACC-v/2(errors) -> virtualErrors/1
  ACC-v/1(u) -> Switch/1
  Switch/1 -> Min/2, Scope1/2  "acc-v"
  lcFlag/1 -> ACC/3(lcFlag), On Delay/1, ACC-v/4(lcFlag)
  ACC/2(errors) -> errors/1
  virtualLeaderStates/1 -> ACC-v/2(leaderStates)
  leaderStates/1 -> ACC/2(leaderStates)
  Bus Creator/1 -> states/1, ACC-v/1(currentStates), ACC/1(currentStates)
  ACC/3(gap) -> gap/1
  Mux1/1 -> Terminator/1
  Vehicle Body 3DOF Single Track/7 -> Mux1/6
  Vehicle Body 3DOF Single Track/6 -> Mux1/5
  Vehicle Body 3DOF Single Track/5 -> Mux1/4
  Vehicle Body 3DOF Single Track/2 -> Mux1/1
  Vehicle Body 3DOF Single Track/3 -> Mux1/2
  Vehicle Body 3DOF Single Track/4 -> Mux1/3
  Vehicle Body 3DOF Single Track/1 -> Bus Selector/1
  Constant/1 -> Vehicle Body 3DOF Single Track/1
  Gain/1 -> Vehicle Body 3DOF Single Track/2, Vehicle Body 3DOF Single Track/3
  ACC/1(u) -> Min/1, Scope1/1  "acc"
  Min/1 -> Signal Specification/1, Scope1/3  "u"
  Bus Selector/1 -> Bus Creator/1  "<X>"
  Bus Selector/3 -> Bus Creator/3  "<Xdot>"

== system gap_generation_platoon/Ld ==
  leaderStates : Inport
  virtualLeaderStates : Inport  Port=2
  lcFlag : Inport  Port=3
  activate ACC-v : Inport  Port=4
  ACC : Subsystem
  ACC-v : Subsystem
  AND : Logic  Inputs=3  IconShape=distinctive  AllPortsSameDT=off  OutDataTypeStr=boolean
  Abs : Abs
  Abs1 : Abs  ZeroCross=off
  Bus Creator : BusCreator  Inputs=4
  Bus Selector : BusSelector  OutputSignals=InertFrm.RearAxl.Disp.X,InertFrm.RearAxl.Disp.Y,InertFrm.RearAxl.Vel.Xdot
  Compare To Constant : simulink/Logic and Bit Operations/Compare To Constant  relop=<=  const=0.5  OutDataTypeStr=boolean
  Compare To Constant1 : simulink/Logic and Bit Operations/Compare To Constant  relop=<=  const=0.5  OutDataTypeStr=boolean
  Constant : Constant  Value=0
  Constant1 : Constant  Value=maxAcceleration+1
  Gain : Gain  Gain=m/2
  Min : MinMax  Inputs=2
  Mux1 : Mux  Inputs=6
  On Delay : powerlib_meascontrol/Logic/On Delay  DelayType=On delay  delay=1  ic=0  Ts=0
      settings: SourceProductName=Simscape Electrical
  Scope : Scope  NumInputPorts=2
  Scope1 : Scope  NumInputPorts=3
  Signal Specification : SignalSpecification  Dimensions=1
  Switch : Switch  Criteria=u2 > Threshold
  Terminator : Terminator
  Transport Delay : TransportDelay
  Triggered Subsystem : Subsystem  TreatAsAtomicUnit=on
  Vehicle Body 3DOF Single Track : autolibshared/Vehicle Body 3DOF Single Track  trackMode=Single (bicycle)  inputMode=External longitudinal forces  frontSteerMode=on  rearSteerMode=off  windMode=off  muMode=off  extFMode=off  extMMode=off  extXo=off  extpsio=off  extxdoto=off  extro=off  extYo=off  extTamb=off  extydoto=off  aMode=2  NF=2  NR=2  m=m  a=lf  b=lr  h=0.35  X_o=x0  xdot_o=vx0  CalphaMode=off  sigmaMode=on  d=0  w=[1.4,1.4]  Cy_f=12e3  Cy_r=11e3  sigma_f=.1  sigma_r=.1  alpha_f_brk=[-.1 .1]  Cy_f_data=[-9e3 9e3]  alpha_r_brk=[-.1 .1]  Cy_r_data=[-9e3 9e3]  Y_o=y0  ydot_o=0  Izz=4000  psi_o=0  r_o=0  Af=2  Cd=.3  Cl=.1  Cpm=.1  beta_w=[0:0.01:0.3]  Cs=[0:0.03:0.9]  Cym=[0:0.01:0.3]  Pabs=101325  Tair=273  g=9.81  mu=1  xdot_tol=.01  Fznom=5000  Fxtire_sat=7e4  Fytire_sat=7e4  longOff=0  latOff=0  vertOff=0  wrapAng=off
      settings: SourceProductName=Powertrain Blockset  SourceProductBaseCode=PW
  states : Outport
  errors : Outport  Port=2
  gap : Outport  Port=3
  virtualErrors : Outport  Port=4
  virtualGap : Outport  Port=5
  gapRequest : Outport  Port=6
  wires:
  Abs1/1 -> Compare To Constant1/1
  Abs/1 -> Compare To Constant/1
  Transport Delay/1 -> Abs/1
  Compare To Constant/1 -> AND/2
  Triggered Subsystem/1(Out1) -> Scope/2, gapRequest/1
  On Delay/1 -> Triggered Subsystem/1(In1), AND/3
  Compare To Constant1/1 -> AND/1, Scope/1
  AND/1 -> Triggered Subsystem/Trigger
  Constant1/1 -> Switch/3
  activate ACC-v/1 -> Switch/2, ACC-v/3(activate)
  Signal Specification/1 -> Gain/1, Bus Creator/4, Abs1/1, Transport Delay/1
  Bus Selector/2 -> Bus Creator/2  "<Y>"
  ACC-v/3(gap) -> virtualGap/1
  ACC-v/2(errors) -> virtualErrors/1
  ACC-v/1(u) -> Switch/1
  Switch/1 -> Min/2, Scope1/2  "acc-v"
  lcFlag/1 -> ACC/3(lcFlag), On Delay/1, ACC-v/4(lcFlag)
  ACC/2(errors) -> errors/1
  virtualLeaderStates/1 -> ACC-v/2(leaderStates)
  leaderStates/1 -> ACC/2(leaderStates)
  Bus Creator/1 -> states/1, ACC-v/1(currentStates), ACC/1(currentStates)
  ACC/3(gap) -> gap/1
  Mux1/1 -> Terminator/1
  Vehicle Body 3DOF Single Track/7 -> Mux1/6
  Vehicle Body 3DOF Single Track/6 -> Mux1/5
  Vehicle Body 3DOF Single Track/5 -> Mux1/4
  Vehicle Body 3DOF Single Track/2 -> Mux1/1
  Vehicle Body 3DOF Single Track/3 -> Mux1/2
  Vehicle Body 3DOF Single Track/4 -> Mux1/3
  Vehicle Body 3DOF Single Track/1 -> Bus Selector/1
  Constant/1 -> Vehicle Body 3DOF Single Track/1
  Gain/1 -> Vehicle Body 3DOF Single Track/2, Vehicle Body 3DOF Single Track/3
  ACC/1(u) -> Min/1, Scope1/1  "acc"
  Min/1 -> Signal Specification/1, Scope1/3  "u"
  Bus Selector/1 -> Bus Creator/1  "<X>"
  Bus Selector/3 -> Bus Creator/3  "<Xdot>"

== system gap_generation_platoon/Lo ==
  leaderStates : Inport
  virtualLeaderStates : Inport  Port=2
  lcFlag : Inport  Port=3
  activate ACC-v : Inport  Port=4
  ACC : Subsystem
  ACC-v : Subsystem
  AND : Logic  Inputs=3  IconShape=distinctive  AllPortsSameDT=off  OutDataTypeStr=boolean
  Abs : Abs
  Abs1 : Abs  ZeroCross=off
  Bus Creator : BusCreator  Inputs=4
  Bus Selector : BusSelector  OutputSignals=InertFrm.RearAxl.Disp.X,InertFrm.RearAxl.Disp.Y,InertFrm.RearAxl.Vel.Xdot
  Compare To Constant : simulink/Logic and Bit Operations/Compare To Constant  relop=<=  const=0.5  OutDataTypeStr=boolean
  Compare To Constant1 : simulink/Logic and Bit Operations/Compare To Constant  relop=<=  const=0.5  OutDataTypeStr=boolean
  Constant : Constant  Value=0
  Constant1 : Constant  Value=maxAcceleration+1
  Gain : Gain  Gain=m/2
  Min : MinMax  Inputs=2
  Mux1 : Mux  Inputs=6
  On Delay : powerlib_meascontrol/Logic/On Delay  DelayType=On delay  delay=1  ic=0  Ts=0
      settings: SourceProductName=Simscape Electrical
  Scope : Scope  NumInputPorts=2
  Scope1 : Scope  NumInputPorts=3
  Signal Specification : SignalSpecification  Dimensions=1
  Switch : Switch  Criteria=u2 > Threshold
  Terminator : Terminator
  Transport Delay : TransportDelay
  Triggered Subsystem : Subsystem  TreatAsAtomicUnit=on
  Vehicle Body 3DOF Single Track : autolibshared/Vehicle Body 3DOF Single Track  trackMode=Single (bicycle)  inputMode=External longitudinal forces  frontSteerMode=on  rearSteerMode=off  windMode=off  muMode=off  extFMode=off  extMMode=off  extXo=off  extpsio=off  extxdoto=off  extro=off  extYo=off  extTamb=off  extydoto=off  aMode=2  NF=2  NR=2  m=m  a=lf  b=lr  h=0.35  X_o=x0  xdot_o=vx0  CalphaMode=off  sigmaMode=on  d=0  w=[1.4,1.4]  Cy_f=12e3  Cy_r=11e3  sigma_f=.1  sigma_r=.1  alpha_f_brk=[-.1 .1]  Cy_f_data=[-9e3 9e3]  alpha_r_brk=[-.1 .1]  Cy_r_data=[-9e3 9e3]  Y_o=y0  ydot_o=0  Izz=4000  psi_o=0  r_o=0  Af=2  Cd=.3  Cl=.1  Cpm=.1  beta_w=[0:0.01:0.3]  Cs=[0:0.03:0.9]  Cym=[0:0.01:0.3]  Pabs=101325  Tair=273  g=9.81  mu=1  xdot_tol=.01  Fznom=5000  Fxtire_sat=7e4  Fytire_sat=7e4  longOff=0  latOff=0  vertOff=0  wrapAng=off
      settings: SourceProductName=Powertrain Blockset  SourceProductBaseCode=PW
  states : Outport
  errors : Outport  Port=2
  gap : Outport  Port=3
  virtualErrors : Outport  Port=4
  virtualGap : Outport  Port=5
  gapRequest : Outport  Port=6
  wires:
  Bus Selector/3 -> Bus Creator/3  "<Xdot>"
  Bus Selector/1 -> Bus Creator/1  "<X>"
  Min/1 -> Scope1/3, Signal Specification/1  "u"
  ACC/1(u) -> Scope1/1, Min/1  "acc"
  Gain/1 -> Vehicle Body 3DOF Single Track/3, Vehicle Body 3DOF Single Track/2
  Constant/1 -> Vehicle Body 3DOF Single Track/1
  Vehicle Body 3DOF Single Track/1 -> Bus Selector/1
  Vehicle Body 3DOF Single Track/4 -> Mux1/3
  Vehicle Body 3DOF Single Track/3 -> Mux1/2
  Vehicle Body 3DOF Single Track/2 -> Mux1/1
  Vehicle Body 3DOF Single Track/5 -> Mux1/4
  Vehicle Body 3DOF Single Track/6 -> Mux1/5
  Vehicle Body 3DOF Single Track/7 -> Mux1/6
  Mux1/1 -> Terminator/1
  ACC/3(gap) -> gap/1
  Bus Creator/1 -> ACC/1(currentStates), ACC-v/1(currentStates), states/1
  leaderStates/1 -> ACC/2(leaderStates)
  virtualLeaderStates/1 -> ACC-v/2(leaderStates)
  ACC/2(errors) -> errors/1
  lcFlag/1 -> ACC-v/4(lcFlag), On Delay/1, ACC/3(lcFlag)
  Switch/1 -> Scope1/2, Min/2  "acc-v"
  ACC-v/1(u) -> Switch/1
  ACC-v/2(errors) -> virtualErrors/1
  ACC-v/3(gap) -> virtualGap/1
  Bus Selector/2 -> Bus Creator/2  "<Y>"
  Signal Specification/1 -> Transport Delay/1, Abs1/1, Bus Creator/4, Gain/1
  activate ACC-v/1 -> ACC-v/3(activate), Switch/2
  Constant1/1 -> Switch/3
  AND/1 -> Triggered Subsystem/Trigger
  Compare To Constant1/1 -> Scope/1, AND/1
  On Delay/1 -> AND/3, Triggered Subsystem/1(In1)
  Triggered Subsystem/1(Out1) -> gapRequest/1, Scope/2
  Compare To Constant/1 -> AND/2
  Transport Delay/1 -> Abs/1
  Abs/1 -> Compare To Constant/1
  Abs1/1 -> Compare To Constant1/1

== system gap_generation_platoon/p1 ==
  leaderStates : Inport
  virtualLeaderStates : Inport  Port=2
  lcFlag : Inport  Port=3
  activate ACC-v : Inport  Port=4
  ACC : Subsystem
  ACC-v : Subsystem
  AND : Logic  IconShape=distinctive  AllPortsSameDT=off  OutDataTypeStr=boolean
  Bus Creator : BusCreator  Inputs=4
  Bus Selector : BusSelector  OutputSignals=InertFrm.RearAxl.Disp.X,InertFrm.RearAxl.Disp.Y,InertFrm.RearAxl.Vel.Xdot
  Constant : Constant  Value=0
  Constant1 : Constant  Value=maxAcceleration+1
  Detect steady state : Subsystem
  Gain : Gain  Gain=m/2
  Min : MinMax  Inputs=2
  Mux1 : Mux  Inputs=6
  On Delay : powerlib_meascontrol/Logic/On Delay  DelayType=On delay  delay=1  ic=0  Ts=0
      settings: SourceProductName=Simscape Electrical
  Scope1 : Scope  NumInputPorts=3
  Signal Specification : SignalSpecification  Dimensions=1
  Switch : Switch  Criteria=u2 > Threshold
  Terminator : Terminator
  Triggered Subsystem : Subsystem  TreatAsAtomicUnit=on
  Vehicle Body 3DOF Single Track : autolibshared/Vehicle Body 3DOF Single Track  trackMode=Single (bicycle)  inputMode=External longitudinal forces  frontSteerMode=on  rearSteerMode=off  windMode=off  muMode=off  extFMode=off  extMMode=off  extXo=off  extpsio=off  extxdoto=off  extro=off  extYo=off  extTamb=off  extydoto=off  aMode=2  NF=2  NR=2  m=m  a=lf  b=lr  h=0.35  X_o=x0  xdot_o=vx0  CalphaMode=off  sigmaMode=on  d=0  w=[1.4,1.4]  Cy_f=12e3  Cy_r=11e3  sigma_f=.1  sigma_r=.1  alpha_f_brk=[-.1 .1]  Cy_f_data=[-9e3 9e3]  alpha_r_brk=[-.1 .1]  Cy_r_data=[-9e3 9e3]  Y_o=y0  ydot_o=0  Izz=4000  psi_o=0  r_o=0  Af=2  Cd=.3  Cl=.1  Cpm=.1  beta_w=[0:0.01:0.3]  Cs=[0:0.03:0.9]  Cym=[0:0.01:0.3]  Pabs=101325  Tair=273  g=9.81  mu=1  xdot_tol=.01  Fznom=5000  Fxtire_sat=7e4  Fytire_sat=7e4  longOff=0  latOff=0  vertOff=0  wrapAng=off
      settings: SourceProductName=Powertrain Blockset  SourceProductBaseCode=PW
  states : Outport
  errors : Outport  Port=2
  gap : Outport  Port=3
  virtualErrors : Outport  Port=4
  virtualGap : Outport  Port=5
  gapRequest : Outport  Port=6
  wires:
  Bus Selector/3 -> Bus Creator/3  "<Xdot>"
  Bus Selector/1 -> Bus Creator/1  "<X>"
  Min/1 -> Scope1/3, Signal Specification/1  "u"
  ACC/1(u) -> Scope1/1, Min/1  "acc"
  Gain/1 -> Vehicle Body 3DOF Single Track/3, Vehicle Body 3DOF Single Track/2
  Constant/1 -> Vehicle Body 3DOF Single Track/1
  Vehicle Body 3DOF Single Track/1 -> Bus Selector/1
  Vehicle Body 3DOF Single Track/4 -> Mux1/3
  Vehicle Body 3DOF Single Track/3 -> Mux1/2
  Vehicle Body 3DOF Single Track/2 -> Mux1/1
  Vehicle Body 3DOF Single Track/5 -> Mux1/4
  Vehicle Body 3DOF Single Track/6 -> Mux1/5
  Vehicle Body 3DOF Single Track/7 -> Mux1/6
  Mux1/1 -> Terminator/1
  ACC/3(gap) -> gap/1
  Bus Creator/1 -> ACC/1(currentStates), ACC-v/1(currentStates), states/1
  leaderStates/1 -> ACC/2(leaderStates)
  virtualLeaderStates/1 -> ACC-v/2(leaderStates)
  ACC/2(errors) -> errors/1, Detect steady state/1(errors)
  lcFlag/1 -> ACC-v/4(lcFlag), On Delay/1, ACC/3(lcFlag)
  Switch/1 -> Scope1/2, Min/2  "acc-v"
  ACC-v/1(u) -> Switch/1
  ACC-v/2(errors) -> Detect steady state/2(virtual errors), virtualErrors/1
  ACC-v/3(gap) -> virtualGap/1
  Bus Selector/2 -> Bus Creator/2  "<Y>"
  Signal Specification/1 -> Bus Creator/4, Gain/1
  activate ACC-v/1 -> Switch/2, ACC-v/3(activate), Detect steady state/3(ACC-v active)
  Constant1/1 -> Switch/3
  AND/1 -> Triggered Subsystem/Trigger
  On Delay/1 -> Triggered Subsystem/1(In1), AND/2
  Triggered Subsystem/1(Out1) -> gapRequest/1
  Detect steady state/1(Out1) -> AND/1
